simulink library "powertrain"  (R2025b)
settings: Solver=VariableStepAuto  StartTime=0.0  StopTime=10.0  RelTol=1e-3
settings Model: Creator=jessi  LastModifiedBy=Admin

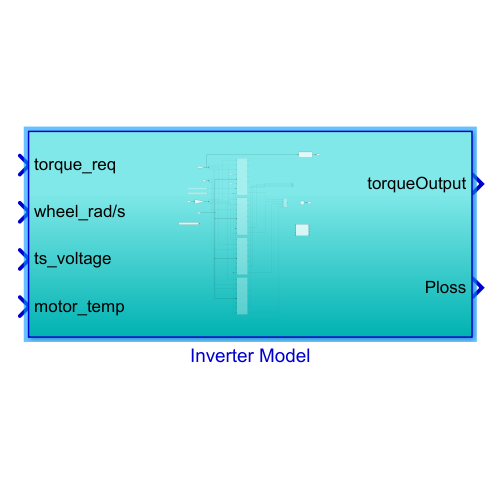
[thumbnail: Simulink's stored preview of the top-level diagram]
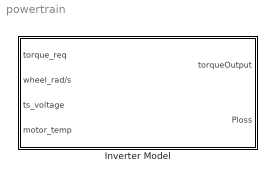
== system powertrain ==
  Inverter Model : Subsystem

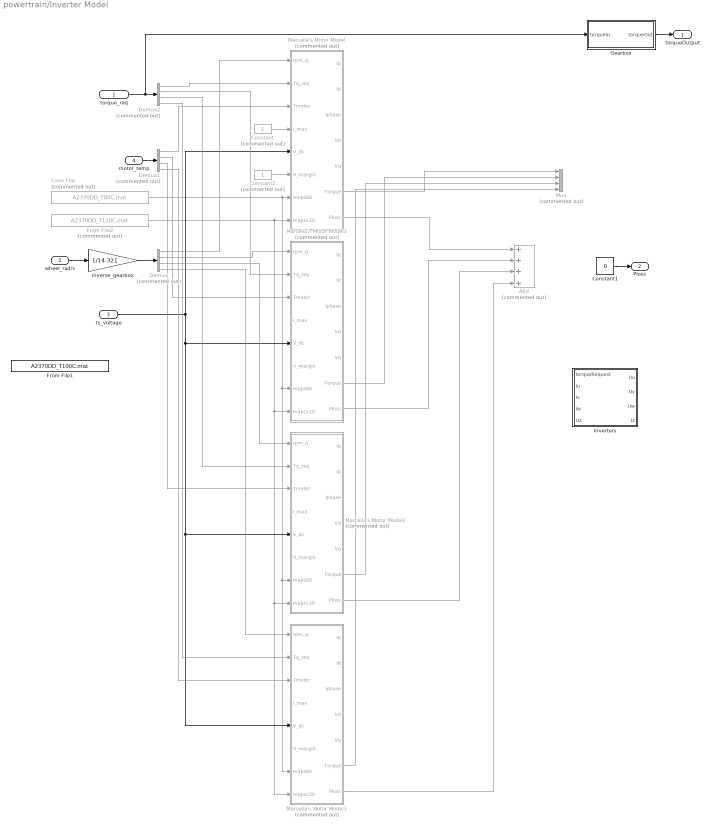
== system powertrain/Inverter Model ==
  torque_req : Inport  Unit=N*m  PortDimensions=4
  wheel_rad/s : Inport  Port=2  Unit=rad/s  PortDimensions=4
  ts_voltage : Inport  Port=3  Unit=V
  motor_temp : Inport  Port=4
  Add : Sum  Commented=on  Inputs=++++
  Constant : Constant  Commented=on
  Constant1 : Constant  Value=0
  Constant2 : Constant  Commented=on
  Demux : Demux  Commented=on
  Demux1 : Demux  Commented=on
  Demux2 : Demux  Commented=on
  From File : FromFile  Commented=on  FileName=A2370DD_T80C.mat  OutDataTypeStr=double  SampleTime=0
  From File1 : FromFile  FileName=A2370DD_T100C.mat  SampleTime=0
  From File2 : FromFile  Commented=on  FileName=A2370DD_T120C.mat  OutDataTypeStr=double  SampleTime=0
  Gearbox : Subsystem
  Inverters : Subsystem
  Marcella's Motor Model : MATLAB Function  Commented=on  TreatAsAtomicUnit=on
  Marcella's Motor Model1 : MATLAB Function  Commented=on  TreatAsAtomicUnit=on
  Marcella's Motor Model2 : MATLAB Function  Commented=on  TreatAsAtomicUnit=on
  Marcella's Motor Model3 : MATLAB Function  Commented=on  TreatAsAtomicUnit=on
  Mux : Mux  Commented=on
  inverse_gearbox : Gain  Gain=1/14.321
  torqueOutput : Outport  Unit=N*m  PortDimensions=4
  Ploss : Outport  Port=2  Unit=A
  wires:
  Gearbox/1(torqueOut) -> torqueOutput/1
  From File2/1 -> Marcella's Motor Model3/8(maps120), Marcella's Motor Model2/8(maps120), Marcella's Motor Model1/8(maps120), Marcella's Motor Model/8(maps120)
  From File/1 -> Marcella's Motor Model3/7(maps80), Marcella's Motor Model2/7(maps80), Marcella's Motor Model1/7(maps80), Marcella's Motor Model/7(maps80)
  Constant/1 -> Marcella's Motor Model/4(I_max)
  Constant2/1 -> Marcella's Motor Model/6(V_margin)
  ts_voltage/1 -> Marcella's Motor Model/5(V_dc), Marcella's Motor Model3/5(V_dc), Marcella's Motor Model2/5(V_dc), Marcella's Motor Model1/5(V_dc)
  Marcella's Motor Model/7(Ploss) -> Add/1
  Marcella's Motor Model1/7(Ploss) -> Add/2
  Marcella's Motor Model2/7(Ploss) -> Add/3
  Marcella's Motor Model3/7(Ploss) -> Add/4
  wheel_rad/s/1 -> inverse_gearbox/1
  Demux/1 -> Marcella's Motor Model/1(rpm_q)
  Demux/2 -> Marcella's Motor Model1/1(rpm_q)
  Demux/3 -> Marcella's Motor Model2/1(rpm_q)
  Demux/4 -> Marcella's Motor Model3/1(rpm_q)
  motor_temp/1 -> Demux1/1
  Demux1/1 -> Marcella's Motor Model/3(Tmotor)
  Demux1/2 -> Marcella's Motor Model1/3(Tmotor)
  Demux1/3 -> Marcella's Motor Model2/3(Tmotor)
  Demux1/4 -> Marcella's Motor Model3/3(Tmotor)
  torque_req/1 -> Gearbox/1(torqueIn), Demux2/1
  Demux2/1 -> Marcella's Motor Model/2(Tq_req)
  Demux2/2 -> Marcella's Motor Model1/2(Tq_req)
  Demux2/3 -> Marcella's Motor Model2/2(Tq_req)
  Demux2/4 -> Marcella's Motor Model3/2(Tq_req)
  Marcella's Motor Model/6(Torque) -> Mux/1
  Marcella's Motor Model1/6(Torque) -> Mux/2
  Marcella's Motor Model2/6(Torque) -> Mux/3
  Marcella's Motor Model3/6(Torque) -> Mux/4
  inverse_gearbox/1 -> Demux/1
  Constant1/1 -> Ploss/1

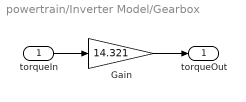
== system powertrain/Inverter Model/Gearbox ==
  torqueIn : Inport  Unit=N*m  PortDimensions=4
  Gain : Gain  Gain=14.321
  torqueOut : Outport  Unit=N*m  PortDimensions=4
  wires:
  torqueIn/1 -> Gain/1
  Gain/1 -> torqueOut/1

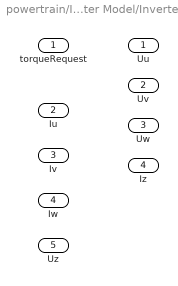
== system powertrain/Inverter Model/Inverters ==
  torqueRequest : Inport
  Iu : Inport  Port=2
  Iv : Inport  Port=3
  Iw : Inport  Port=4
  Uz : Inport  Port=5
  Uu : Outport
  Uv : Outport  Port=2
  Uw : Outport  Port=3
  Iz : Outport  Port=4

== matlab function powertrain/Inverter Model/Marcella's Motor Model1 ==
  data: rpm_q input; Tq_req input; Tmotor input; I_max input; V_dc input; V_margin input; maps80 input; maps120 input; Iq output; Id output; Iphase output; Vd output; Vq output; Torque output; Ploss output
function [Iq, Id, Iphase, Vd, Vq, Torque, Ploss]= fcn(rpm_q,Tq_req, Tmotor, I_max, V_dc, V_margin, maps80, maps120)
    limits = struct();
    limits.I_max = I_max;
    limits.V_dc = V_dc;
    limits.V_margin = V_margin;
    out = motor_map_model_function(rpm_q, Tq_req, Tmotor, maps80, maps120, limits);
    Iq = out.Iq;
    Id = out.Id;
    Iphase = out.Iphase;
    Vd = out.Vd;
    Vq = out.Vq;
    Torque = out.Torque;
    Ploss = out.Ploss;
end

== matlab function powertrain/Inverter Model/Marcella's Motor Model ==
  data: rpm_q input; Tq_req input; Tmotor input; I_max input; V_dc input; V_margin input; maps80 input; maps120 input; Iq output; Id output; Iphase output; Vd output; Vq output; Torque output; Ploss output
function [Iq, Id, Iphase, Vd, Vq, Torque, Ploss]= fcn(rpm_q,Tq_req, Tmotor, I_max, V_dc, V_margin, maps80, maps120)
    limits = struct();
    limits.I_max = I_max;
    limits.V_dc = V_dc;
    limits.V_margin = V_margin;
    out = motor_map_model_function(rpm_q, Tq_req, Tmotor, maps80, maps120, limits);
    Iq = out.Iq;
    Id = out.Id;
    Iphase = out.Iphase;
    Vd = out.Vd;
    Vq = out.Vq;
    Torque = out.Torque;
    Ploss = out.Ploss;
end

== matlab function powertrain/Inverter Model/Marcella's Motor Model2 ==
  data: rpm_q input; Tq_req input; Tmotor input; I_max input; V_dc input; V_margin input; maps80 input; maps120 input; Iq output; Id output; Iphase output; Vd output; Vq output; Torque output; Ploss output
function [Iq, Id, Iphase, Vd, Vq, Torque, Ploss]= fcn(rpm_q,Tq_req, Tmotor, I_max, V_dc, V_margin, maps80, maps120)
    limits = struct();
    limits.I_max = I_max;
    limits.V_dc = V_dc;
    limits.V_margin = V_margin;
    out = motor_map_model_function(rpm_q, Tq_req, Tmotor, maps80, maps120, limits);
    Iq = out.Iq;
    Id = out.Id;
    Iphase = out.Iphase;
    Vd = out.Vd;
    Vq = out.Vq;
    Torque = out.Torque;
    Ploss = out.Ploss;
end

== matlab function powertrain/Inverter Model/Marcella's Motor Model3 ==
  data: rpm_q input; Tq_req input; Tmotor input; I_max input; V_dc input; V_margin input; maps80 input; maps120 input; Iq output; Id output; Iphase output; Vd output; Vq output; Torque output; Ploss output
function [Iq, Id, Iphase, Vd, Vq, Torque, Ploss]= fcn(rpm_q,Tq_req, Tmotor, I_max, V_dc, V_margin, maps80, maps120)
    limits = struct();
    limits.I_max = I_max;
    limits.V_dc = V_dc;
    limits.V_margin = V_margin;
    out = motor_map_model_function(rpm_q, Tq_req, Tmotor, maps80, maps120, limits);
    Iq = out.Iq;
    Id = out.Id;
    Iphase = out.Iphase;
    Vd = out.Vd;
    Vq = out.Vq;
    Torque = out.Torque;
    Ploss = out.Ploss;
end
